simulink model "Poject_PilotInLoop_Beech_99_Linear_Transfer_Function_Bank"  (R2018b)
settings: Solver=VariableStepAuto  StartTime=0.0  StopTime=100  RelTol=1e-3
InitFcn:
  | Initial_Data_Bank
StopFcn:
  | PilotInLoopPlotsBank
values from neighbouring files (symbols this model uses):
  Kp = 1    [Initial_Data_Bank.m]    (also in PilotInLoopBank.m)
  LdelA = 17.1510    (= 17.151)    [Initial_Data_Bank.m]    (also in PilotInLoopBank.m)
  Lp = -2.81    [Initial_Data_Bank.m]    (also in PilotInLoopBank.m)
  taw = 0.1    [Initial_Data_Bank.m]    (also in PilotInLoopBank.m)
  TI = 0.2    [Initial_Data_Bank.m]    (also in PilotInLoopBank.m)
  TL = 0.4    [Initial_Data_Bank.m]    (also in PilotInLoopBank.m)
  TN = 0.1    [Initial_Data_Bank.m]    (also in PilotInLoopBank.m)
settings Model: Creator=User  LastModifiedBy=User

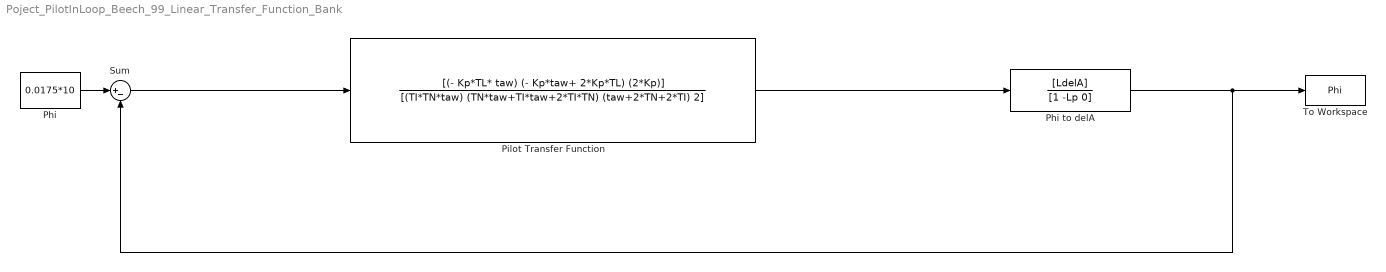
== system Poject_PilotInLoop_Beech_99_Linear_Transfer_Function_Bank ==
  Phi : Constant  Value=0.0175*10
  Phi to delA : TransferFcn  Numerator=[LdelA]  Denominator=[1 -Lp 0]
  Pilot Transfer Function : TransferFcn  Numerator=[(- Kp*TL* taw) (- Kp*taw+ 2*Kp*TL) (2*Kp)]  Denominator=[(TI*TN*taw) (TN*taw+TI*taw+2*TI*TN) (taw+2*TN+2*TI) 2]
  Sum : Sum  Inputs=|+-
  To Workspace : ToWorkspace  VariableName=Phi  SaveFormat=Timeseries  SampleTime=-1
  wires:
  Pilot Transfer Function/1 -> Phi to delA/1
  Phi to delA/1 -> To Workspace/1, Sum/2
  Phi/1 -> Sum/1
  Sum/1 -> Pilot Transfer Function/1
